simulink model "Lab7_1811"  (R2021b)
settings: Solver=VariableStepAuto  StartTime=0.0  StopTime=10.0  RelTol=1e-3
values from neighbouring files (symbols this model uses):
  a = 1/( 2/norm(r0) - dot(v0,v0)/mu_E )    [Excercise1_2223.m]    (also in Excercise2_2223.m; Lab08_script.m = 42164; Lab7_script.m = 16733.65; Lab7_scriptscalar.m = 16733.65)
  A0 = eye(3)    [Lab08_script.m]    (also in Lab7_script.m; Lab7_scriptscalar.m; Lab_GG.m)
  Area_mb = diag([A1 A2 A3 A4 A5 A6])    [Lab08_script.m]    (also in Lab7_script.m)
  e = horizonsresults(:,2)    [Ex3-5.m]    (also in Excercise1_2223.m = 1/mu_E*cross(v,h)-r./vecnorm(r,2,2); Lab08_script.m = 0; Lab7_script.m = 0.1976; Lab7_scriptscalar.m = 0.1976)
  epsilon = (vecnorm(v,2,2)).^2/2-mu_E./vecnorm(r,2,2)    [Excercise1_2223.m]    (also in Lab08_script.m = deg2rad(23.45); Lab7_script.m = deg2rad(23.45); Lab7_scriptscalar.m = deg2rad(23.45))
  I = [Ix 0 0; 0 Iy 0; 0 0 Iz]    [Lab08_script.m]    (also in Lab7_script.m; Lab7_scriptscalar.m; Lab_GG.m)
  i = horizonsresults(:,3)    [Ex3-5.m]    (also in Lab08_script.m = deg2rad(0); Lab7_script.m = deg2rad(60); Lab7_scriptscalar.m = deg2rad(60); ex3_Lambert.m = kep_arr_M(3))
  I_inv = inv(I)    [Lab08_script.m]    (also in Lab7_script.m; Lab7_scriptscalar.m; Lab_GG.m)
  n = 10    [Chapter3.m]    (also in Lab08_script.m = sqrt(mu_E/(a^3)); Lab7_script.m = sqrt(mu_E/(a^3)); Lab7_scriptscalar.m = sqrt(mu_E/(a^3)); Lab_GG.m = sqrt(mu_E/( R_E+r_orbit)^3))
  N_b_mb = [n1'; n2'; n3'; n4'; n5'; n6']    [Lab08_script.m]    (also in Lab7_script.m)
  n_sun = 2*pi/T_sun    (= 1.99238499086e-07)    [Lab08_script.m]    (also in Lab7_script.m; Lab7_scriptscalar.m)
  r_mb = [base/2 0 0; 0 base/2 0; 0 0 height/2; -base/2 0 0; 0 -base/2 0; 0 0 -height/2]    [Lab08_script.m]
  rho_d_mb = 0.1    [Lab08_script.m]    (also in Lab7_script.m; Lab7_scriptscalar.m)
  rho_s_mb = 0.5    [Lab08_script.m]    (also in Lab7_script.m; Lab7_scriptscalar.m)
  Rs = astroConstants(2)    [Lab08_script.m]    (also in Lab7_script.m; Lab7_scriptscalar.m)
  theta0 = deg2rad(0)    [Lab08_script.m]    (also in Lab7_script.m = deg2rad(230); Lab7_scriptscalar.m = deg2rad(230))
  v1 = [Y1(:,4) Y1(:,5) Y1(:,6)]    [Excercise2_2223.m]    (also in Lab08_script.m = [0 1 -1]'; Lab7_script.m = [0 1 -1]'; Lab7_scriptscalar.m = [0 1 -1]'; Lab_GG.m = [0 1 -1]')
  v2 = [Y2(:,4) Y2(:,5) Y2(:,6)]    [Excercise2_2223.m]    (also in Lab08_script.m = [-1 0 1]'; Lab7_script.m = [-1 0 1]'; Lab7_scriptscalar.m = [-1 0 1]'; Lab_GG.m = [-1 0 1]')
  v3 = [1 -1 0]'    [Lab08_script.m]    (also in Lab7_script.m; Lab7_scriptscalar.m; Lab_GG.m)
libraries: matrix_library x7
settings Model: Creator=sferl  LastModifiedBy=sferl

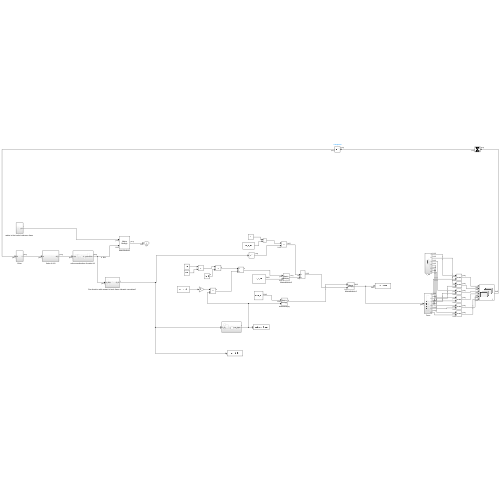
[thumbnail: Simulink's stored preview of the top-level diagram]
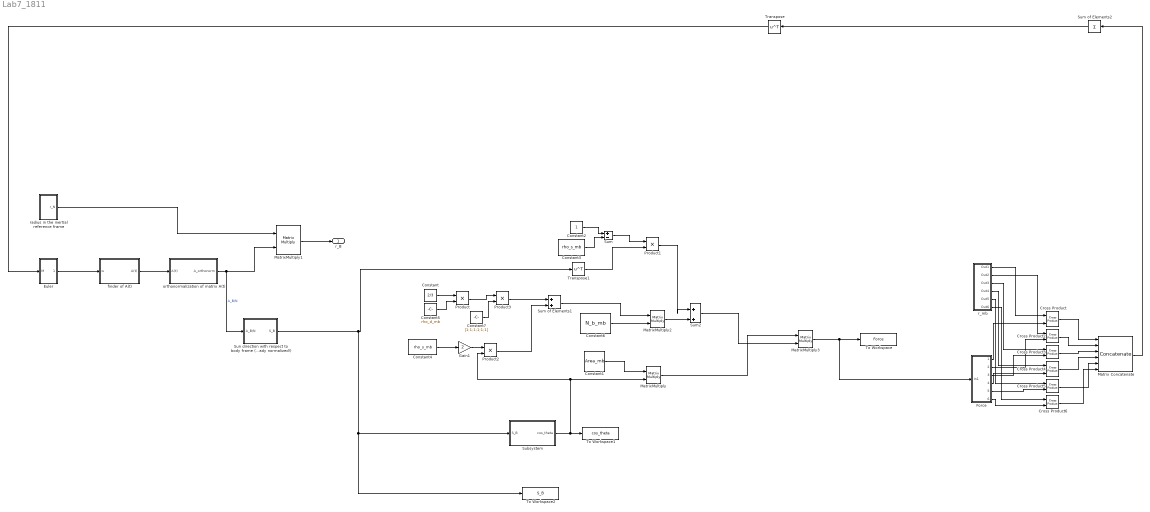
== system Lab7_1811 ==
  Constant : Constant  Value=2/3
  Constant1 : Constant  Value=Area_mb
  Constant2 : Constant
  Constant3 : Constant  Value=rho_s_mb
  Constant4 : Constant  Value=rho_s_mb
  Constant5 : Constant  Value=rho_d_mb
  Constant6 : Constant  Value=N_b_mb
  Constant7 : Constant  Value=[1;1;1;1;1;1]
  Cross Product{,2..6} (6 alike) : matrix_library/Cross Product
      settings: SourceProductBaseCode=SL
  Euler : Subsystem
  Force : Subsystem
  Gain1 : Gain  Gain=2
  Matrix Concatenate : Concatenate  NumInputs=6  Mode=Multidimensional array
  MatrixMultiply{,1..3} (4 alike) : Product  Multiplication=Matrix(*)
  Product{,1..3} (4 alike) : Product
  Subsystem : Subsystem
  Sum : Sum  Inputs=+-
  Sum of Elements1 : Sum
  Sum of Elements2 : Sum  Inputs=+  CollapseMode=Specified dimension
  Sum2 : Sum  Inputs=|++
  Sun direction with respect to body frame (already normalized!) : Subsystem
  To Workspace : ToWorkspace  VariableName=Force  SaveFormat=Timeseries  SampleTime=-1
  To Workspace1 : ToWorkspace  VariableName=cos_theta  SampleTime=-1
  To Workspace2 : ToWorkspace  VariableName=S_B  SampleTime=-1
  Transpose : Math  Operator=transpose  SaturateOnIntegerOverflow=on
  Transpose1 : Math  Operator=transpose  SaturateOnIntegerOverflow=on
  finder of A(t) : Subsystem
  orthonormalization of matrix A(t) : Subsystem
  r_mb : Subsystem
  radius in the inertial reference frame : Subsystem
  r_B : Outport
  wires:
  MatrixMultiply1/1 -> r_B/1
  finder of A(t)/1(A(t)) -> orthonormalization of matrix A(t)/1(A(t))
  orthonormalization of matrix A(t)/1(A_orthonorm) -> Sun direction with respect to body frame (already normalized!)/1(A_B/N), MatrixMultiply1/2  "A_B/N"
  Constant1/1 -> MatrixMultiply/1
  Subsystem/1(cos_theta) -> Product2/2, MatrixMultiply/2, To Workspace1/1
  Constant2/1 -> Sum/1
  Constant3/1 -> Sum/2
  Sum/1 -> Product1/1
  Constant4/1 -> Gain1/1
  Gain1/1 -> Product2/1
  Constant6/1 -> MatrixMultiply2/2
  MatrixMultiply2/1 -> Sum2/2
  Product1/1 -> Sum2/1
  Sum2/1 -> MatrixMultiply3/2
  Transpose1/1 -> Product1/2
  Product/1 -> Product3/1
  Sum of Elements1/1 -> MatrixMultiply2/1
  Constant/1 -> Product/1
  Constant5/1 -> Product/2
  Constant7/1 -> Product3/2
  Product3/1 -> Sum of Elements1/1
  radius in the inertial reference frame/1(r_N) -> MatrixMultiply1/1
  Euler/1(Output1) -> finder of A(t)/1(w)
  Sun direction with respect to body frame (already normalized!)/1(S_B) -> Transpose1/1, Subsystem/1(S_B), To Workspace2/1
  Product2/1 -> Sum of Elements1/2
  MatrixMultiply/1 -> MatrixMultiply3/1
  Cross Product6/1 -> Matrix Concatenate/6
  Cross Product4/1 -> Matrix Concatenate/4
  Cross Product5/1 -> Matrix Concatenate/5
  Cross Product3/1 -> Matrix Concatenate/3
  Matrix Concatenate/1 -> Sum of Elements2/1
  MatrixMultiply3/1 -> Force/1(In1), To Workspace/1
  Cross Product/1 -> Matrix Concatenate/1
  Cross Product2/1 -> Matrix Concatenate/2
  Sum of Elements2/1 -> Transpose/1
  Transpose/1 -> Euler/1(M)
  r_mb/1(Out1) -> Cross Product/1
  r_mb/2(Out2) -> Cross Product2/1
  r_mb/3(Out3) -> Cross Product3/1
  r_mb/4(Out4) -> Cross Product4/1
  r_mb/5(Out5) -> Cross Product5/1
  r_mb/6(Out6) -> Cross Product6/1
  Force/1(Out1) -> Cross Product/2
  Force/2(Out2) -> Cross Product2/2
  Force/3(Out3) -> Cross Product3/2
  Force/4(Out4) -> Cross Product4/2
  Force/5(Out5) -> Cross Product5/2
  Force/6(Out6) -> Cross Product6/2

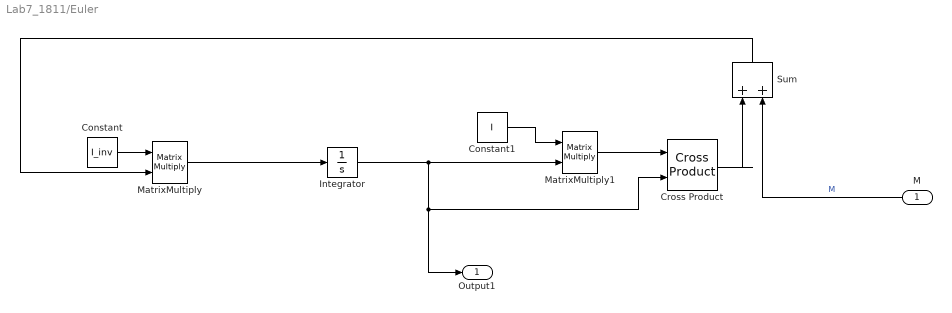
== system Lab7_1811/Euler ==
  M : Inport
  Constant : Constant  Value=I_inv
  Constant1 : Constant  Value=I
  Cross Product : matrix_library/Cross Product
      settings: SourceProductBaseCode=SL
  Integrator : Integrator
  MatrixMultiply : Product  Multiplication=Matrix(*)
  MatrixMultiply1 : Product  Multiplication=Matrix(*)
  Sum : Sum  Inputs=|++
  Output1 : Outport
  wires:
  M/1 -> Sum/2  "M"
  Constant/1 -> MatrixMultiply/1
  MatrixMultiply/1 -> Integrator/1
  Integrator/1 -> Output1/1, Cross Product/2, MatrixMultiply1/2
  Constant1/1 -> MatrixMultiply1/1
  MatrixMultiply1/1 -> Cross Product/1
  Cross Product/1 -> Sum/1
  Sum/1 -> MatrixMultiply/2

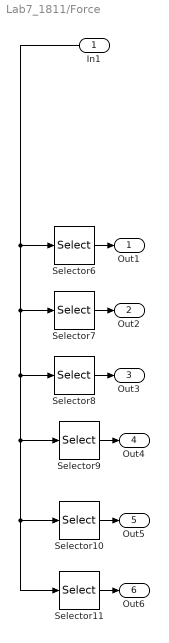
== system Lab7_1811/Force ==
  In1 : Inport
  Selector10 : Selector  NumberOfDimensions=2  InputPortWidth=3  IndexOptions=Starting index (dialog),Starting index (dialog)  Indices=5,1  OutputSizes=1,3
  Selector11 : Selector  NumberOfDimensions=2  InputPortWidth=3  IndexOptions=Starting index (dialog),Starting index (dialog)  Indices=6,1  OutputSizes=1,3
  Selector6 : Selector  NumberOfDimensions=2  InputPortWidth=3  IndexOptions=Starting index (dialog),Starting index (dialog)  Indices=1,1  OutputSizes=1,3
  Selector7 : Selector  NumberOfDimensions=2  InputPortWidth=3  IndexOptions=Starting index (dialog),Starting index (dialog)  Indices=2,1  OutputSizes=1,3
  Selector8 : Selector  NumberOfDimensions=2  InputPortWidth=3  IndexOptions=Starting index (dialog),Starting index (dialog)  Indices=3,1  OutputSizes=1,3
  Selector9 : Selector  NumberOfDimensions=2  InputPortWidth=3  IndexOptions=Starting index (dialog),Starting index (dialog)  Indices=4,1  OutputSizes=1,3
  Out1 : Outport
  Out2 : Outport  Port=2
  Out3 : Outport  Port=3
  Out4 : Outport  Port=4
  Out5 : Outport  Port=5
  Out6 : Outport  Port=6
  wires:
  Selector7/1 -> Out2/1
  Selector6/1 -> Out1/1
  In1/1 -> Selector11/1, Selector10/1, Selector9/1, Selector8/1, Selector7/1, Selector6/1
  Selector9/1 -> Out4/1
  Selector11/1 -> Out6/1
  Selector10/1 -> Out5/1
  Selector8/1 -> Out3/1

== system Lab7_1811/Subsystem ==
  S_B : Inport
  Constant : Constant  Value=N_b_mb
  MatrixMultiply : Product  Multiplication=Matrix(*)
  cos_theta : Outport
  wires:
  Constant/1 -> MatrixMultiply/1
  MatrixMultiply/1 -> cos_theta/1
  S_B/1 -> MatrixMultiply/2

== system Lab7_1811/Sun direction with respect to body frame (already normalized!) ==
  A_B/N : Inport
  Constant7 : Constant  Value=1/Rs
  MatrixMultiply : Product  Multiplication=Matrix(*)
  Product5 : Product
  S_N : Subsystem
  S_B : Outport
  wires:
  S_N/1(Out1) -> MatrixMultiply/2
  A_B/N/1 -> MatrixMultiply/1
  Constant7/1 -> Product5/1
  MatrixMultiply/1 -> Product5/2
  Product5/1 -> S_B/1

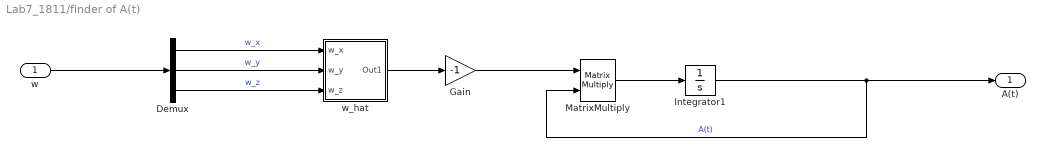
== system Lab7_1811/finder of A(t) ==
  w : Inport
  Demux : Demux  Outputs=3
  Gain : Gain  Gain=-1
  Integrator1 : Integrator  InitialCondition=A0
  MatrixMultiply : Product  Multiplication=Matrix(*)
  w_hat : Subsystem
  A(t) : Outport
  wires:
  w/1 -> Demux/1
  Gain/1 -> MatrixMultiply/1
  Integrator1/1 -> A(t)/1, MatrixMultiply/2  "A(t)"
  w_hat/1(Out1) -> Gain/1
  Demux/3 -> w_hat/3(w_z)  "w_z"
  Demux/2 -> w_hat/2(w_y)  "w_y"
  Demux/1 -> w_hat/1(w_x)  "w_x"
  MatrixMultiply/1 -> Integrator1/1

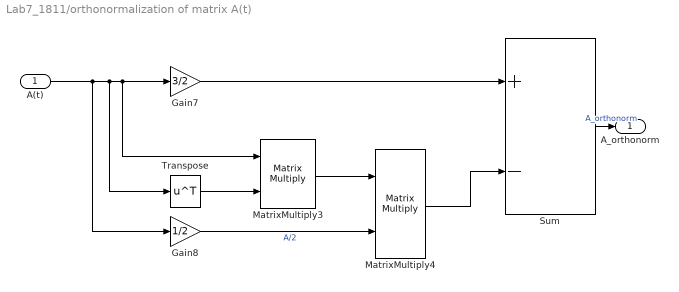
== system Lab7_1811/orthonormalization of matrix A(t) ==
  A(t) : Inport
  Gain7 : Gain  Gain=3/2
  Gain8 : Gain  Gain=1/2
  MatrixMultiply3 : Product  Multiplication=Matrix(*)
  MatrixMultiply4 : Product  Multiplication=Matrix(*)
  Sum : Sum  Inputs=+-
  Transpose : Math  Operator=transpose  SaturateOnIntegerOverflow=on
  A_orthonorm : Outport
  wires:
  Transpose/1 -> MatrixMultiply3/2
  MatrixMultiply4/1 -> Sum/2
  MatrixMultiply3/1 -> MatrixMultiply4/1
  Gain7/1 -> Sum/1
  Gain8/1 -> MatrixMultiply4/2  "A/2"
  A(t)/1 -> Gain8/1, Transpose/1, MatrixMultiply3/1, Gain7/1
  Sum/1 -> A_orthonorm/1  "A_orthonorm"

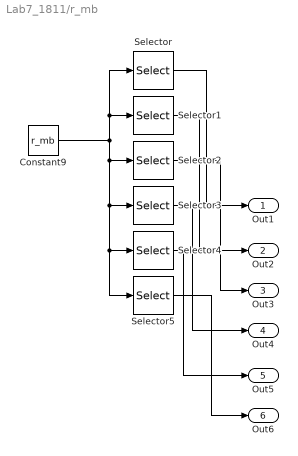
== system Lab7_1811/r_mb ==
  Constant9 : Constant  Value=r_mb
  Selector : Selector  NumberOfDimensions=2  InputPortWidth=3  IndexOptions=Starting index (dialog),Starting index (dialog)  Indices=1,1  OutputSizes=1,3
  Selector1 : Selector  NumberOfDimensions=2  InputPortWidth=3  IndexOptions=Starting index (dialog),Starting index (dialog)  Indices=2,1  OutputSizes=1,3
  Selector2 : Selector  NumberOfDimensions=2  InputPortWidth=3  IndexOptions=Starting index (dialog),Starting index (dialog)  Indices=3,1  OutputSizes=1,3
  Selector3 : Selector  NumberOfDimensions=2  InputPortWidth=3  IndexOptions=Starting index (dialog),Starting index (dialog)  Indices=4,1  OutputSizes=1,3
  Selector4 : Selector  NumberOfDimensions=2  InputPortWidth=3  IndexOptions=Starting index (dialog),Starting index (dialog)  Indices=5,1  OutputSizes=1,3
  Selector5 : Selector  NumberOfDimensions=2  InputPortWidth=3  IndexOptions=Starting index (dialog),Starting index (dialog)  Indices=6,1  OutputSizes=1,3
  Out1 : Outport
  Out2 : Outport  Port=2
  Out3 : Outport  Port=3
  Out4 : Outport  Port=4
  Out5 : Outport  Port=5
  Out6 : Outport  Port=6
  wires:
  Selector4/1 -> Out5/1
  Constant9/1 -> Selector2/1, Selector5/1, Selector4/1, Selector3/1, Selector1/1, Selector/1
  Selector2/1 -> Out3/1
  Selector1/1 -> Out2/1
  Selector/1 -> Out1/1
  Selector3/1 -> Out4/1
  Selector5/1 -> Out6/1

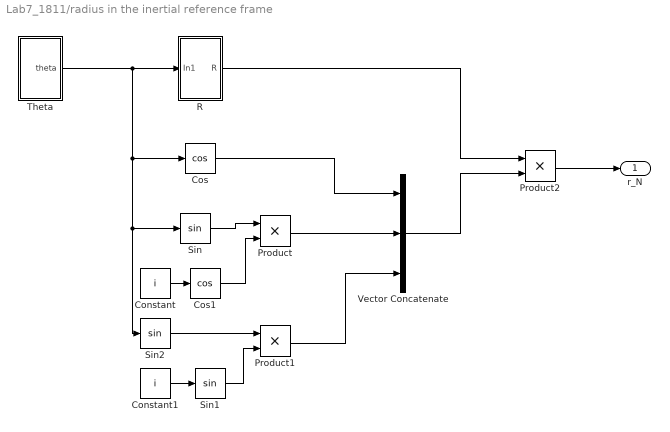
== system Lab7_1811/radius in the inertial reference frame ==
  Constant : Constant  Value=i
  Constant1 : Constant  Value=i
  Cos : Trigonometry  Operator=cos
  Cos1 : Trigonometry  Operator=cos
  Product : Product
  Product1 : Product
  Product2 : Product
  R : Subsystem
  Sin : Trigonometry
  Sin1 : Trigonometry
  Sin2 : Trigonometry
  Theta : Subsystem
  Vector Concatenate : Concatenate  NumInputs=3
  r_N : Outport
  wires:
  Cos/1 -> Vector Concatenate/1
  Theta/1(theta) -> Sin2/1, Sin/1, Cos/1, R/1(In1)
  Constant/1 -> Cos1/1
  Product1/1 -> Vector Concatenate/3
  Sin1/1 -> Product1/2
  Cos1/1 -> Product/2
  R/1(R) -> Product2/1
  Product/1 -> Vector Concatenate/2
  Vector Concatenate/1 -> Product2/2
  Constant1/1 -> Sin1/1
  Sin/1 -> Product/1
  Sin2/1 -> Product1/1
  Product2/1 -> r_N/1

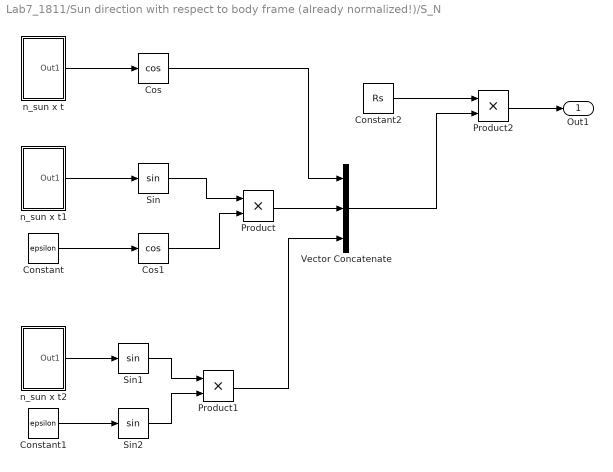
== system Lab7_1811/Sun direction with respect to body frame (already normalized!)/S_N ==
  Constant : Constant  Value=epsilon
  Constant1 : Constant  Value=epsilon
  Constant2 : Constant  Value=Rs
  Cos : Trigonometry  Operator=cos
  Cos1 : Trigonometry  Operator=cos
  Product : Product
  Product1 : Product
  Product2 : Product
  Sin : Trigonometry
  Sin1 : Trigonometry
  Sin2 : Trigonometry
  Vector Concatenate : Concatenate  NumInputs=3
  n_sun x t : Subsystem
  n_sun x t1 : Subsystem
  n_sun x t2 : Subsystem
  Out1 : Outport
  wires:
  n_sun x t2/1(Out1) -> Sin1/1
  Vector Concatenate/1 -> Product2/2
  Sin2/1 -> Product1/2
  Sin/1 -> Product/1
  n_sun x t1/1(Out1) -> Sin/1
  Product1/1 -> Vector Concatenate/3
  Constant2/1 -> Product2/1
  Cos/1 -> Vector Concatenate/1
  Cos1/1 -> Product/2
  Product/1 -> Vector Concatenate/2
  n_sun x t/1(Out1) -> Cos/1
  Constant1/1 -> Sin2/1
  Sin1/1 -> Product1/1
  Constant/1 -> Cos1/1
  Product2/1 -> Out1/1

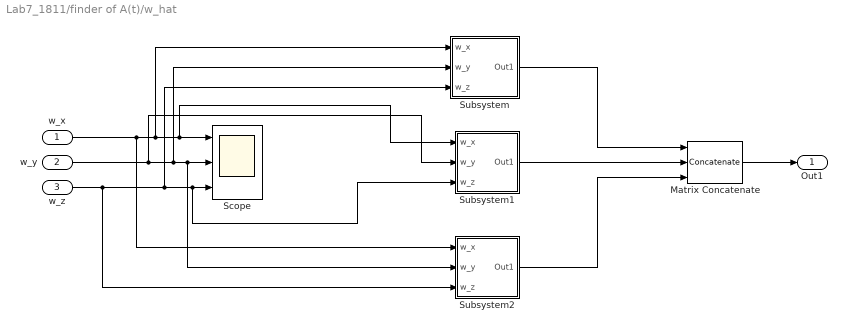
== system Lab7_1811/finder of A(t)/w_hat ==
  w_x : Inport
  w_y : Inport  Port=2
  w_z : Inport  Port=3
  Matrix Concatenate : Concatenate  NumInputs=3  Mode=Multidimensional array  ConcatenateDimension=2
  Scope : Scope  NumInputPorts=3
  Subsystem : Subsystem
  Subsystem1 : Subsystem
  Subsystem2 : Subsystem
  Out1 : Outport
  wires:
  w_y/1 -> Subsystem1/2(w_y), Subsystem/2(w_y), Subsystem2/2(w_y), Scope/2
  w_z/1 -> Subsystem2/3(w_z), Subsystem/3(w_z), Subsystem1/3(w_z), Scope/3
  w_x/1 -> Subsystem2/1(w_x), Subsystem/1(w_x), Subsystem1/1(w_x), Scope/1
  Subsystem2/1(Out1) -> Matrix Concatenate/3
  Subsystem1/1(Out1) -> Matrix Concatenate/2
  Subsystem/1(Out1) -> Matrix Concatenate/1
  Matrix Concatenate/1 -> Out1/1

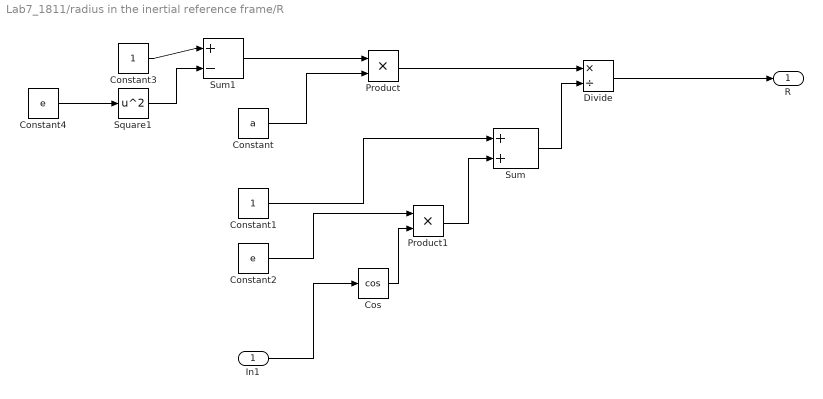
== system Lab7_1811/radius in the inertial reference frame/R ==
  In1 : Inport
  Constant : Constant  Value=a
  Constant1 : Constant
  Constant2 : Constant  Value=e
  Constant3 : Constant
  Constant4 : Constant  Value=e
  Cos : Trigonometry  Operator=cos
  Divide : Product  Inputs=*/
  Product : Product
  Product1 : Product
  Square1 : Math  Operator=square  SaturateOnIntegerOverflow=on
  Sum : Sum  Inputs=|++
  Sum1 : Sum  Inputs=|+-
  R : Outport
  wires:
  Sum/1 -> Divide/2
  Constant1/1 -> Sum/1
  Square1/1 -> Sum1/2
  Product1/1 -> Sum/2
  Constant2/1 -> Product1/1
  Constant/1 -> Product/2
  Divide/1 -> R/1
  Cos/1 -> Product1/2
  Sum1/1 -> Product/1
  In1/1 -> Cos/1
  Constant4/1 -> Square1/1
  Constant3/1 -> Sum1/1
  Product/1 -> Divide/1

== system Lab7_1811/radius in the inertial reference frame/Theta ==
  Denominator : Subsystem
  Divide : Product  Inputs=*/
  Integrator : Integrator  InitialCondition=theta0
  Numerator : Subsystem
  theta : Outport
  wires:
  Numerator/1(Out1) -> Divide/1
  Denominator/1(Output) -> Divide/2
  Integrator/1 -> theta/1, Numerator/1(In1)
  Divide/1 -> Integrator/1

== system Lab7_1811/Sun direction with respect to body frame (already normalized!)/S_N/n_sun x t ==
  Clock : Clock
  Constant : Constant  Value=n_sun
  Product : Product
  Out1 : Outport
  wires:
  Constant/1 -> Product/1
  Clock/1 -> Product/2
  Product/1 -> Out1/1

== system Lab7_1811/Sun direction with respect to body frame (already normalized!)/S_N/n_sun x t1 ==
  Clock : Clock
  Constant : Constant  Value=n_sun
  Product : Product
  Out1 : Outport
  wires:
  Product/1 -> Out1/1
  Clock/1 -> Product/2
  Constant/1 -> Product/1

== system Lab7_1811/Sun direction with respect to body frame (already normalized!)/S_N/n_sun x t2 ==
  Clock : Clock
  Constant : Constant  Value=n_sun
  Product : Product
  Out1 : Outport
  wires:
  Constant/1 -> Product/1
  Clock/1 -> Product/2
  Product/1 -> Out1/1

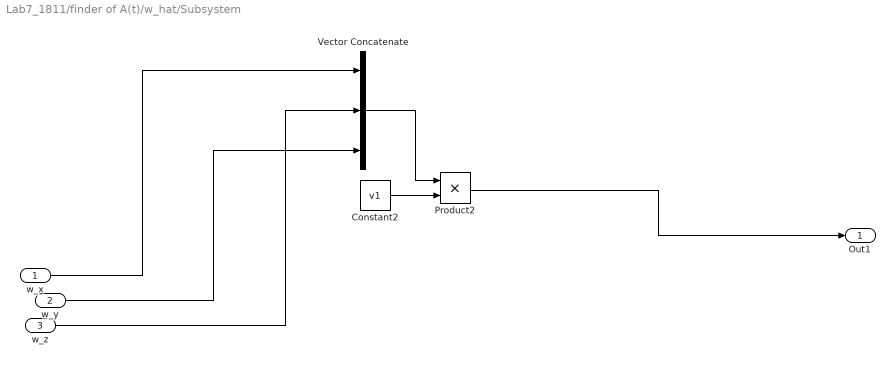
== system Lab7_1811/finder of A(t)/w_hat/Subsystem ==
  w_x : Inport
  w_y : Inport  Port=2
  w_z : Inport  Port=3
  Constant2 : Constant  Value=v1
  Product2 : Product
  Vector Concatenate : Concatenate  NumInputs=3
  Out1 : Outport
  wires:
  Product2/1 -> Out1/1
  Vector Concatenate/1 -> Product2/1
  Constant2/1 -> Product2/2
  w_x/1 -> Vector Concatenate/1
  w_z/1 -> Vector Concatenate/2
  w_y/1 -> Vector Concatenate/3

== system Lab7_1811/finder of A(t)/w_hat/Subsystem1 ==
  w_x : Inport
  w_y : Inport  Port=2
  w_z : Inport  Port=3
  Constant4 : Constant  Value=v2
  Product4 : Product
  Vector Concatenate2 : Concatenate  NumInputs=3
  Out1 : Outport
  wires:
  Constant4/1 -> Product4/2
  Vector Concatenate2/1 -> Product4/1
  Product4/1 -> Out1/1
  w_x/1 -> Vector Concatenate2/3
  w_y/1 -> Vector Concatenate2/2
  w_z/1 -> Vector Concatenate2/1

== system Lab7_1811/finder of A(t)/w_hat/Subsystem2 ==
  w_x : Inport
  w_y : Inport  Port=2
  w_z : Inport  Port=3
  Constant3 : Constant  Value=v3
  Product3 : Product
  Vector Concatenate1 : Concatenate  NumInputs=3
  Out1 : Outport
  wires:
  Product3/1 -> Out1/1
  Constant3/1 -> Product3/2
  w_y/1 -> Vector Concatenate1/1
  Vector Concatenate1/1 -> Product3/1
  w_x/1 -> Vector Concatenate1/2
  w_z/1 -> Vector Concatenate1/3

== system Lab7_1811/radius in the inertial reference frame/Theta/Denominator ==
  Constant3 : Constant
  Constant5 : Constant  Value=3/2
  Power : Math  Operator=pow  SaturateOnIntegerOverflow=on
  Square1 : Math  Operator=square  SaturateOnIntegerOverflow=on
  Sum1 : Sum  Inputs=|+-
  eccentricity : Constant  Value=e
  Output : Outport
  wires:
  Constant3/1 -> Sum1/1
  eccentricity/1 -> Square1/1
  Sum1/1 -> Power/1
  Square1/1 -> Sum1/2
  Constant5/1 -> Power/2
  Power/1 -> Output/1

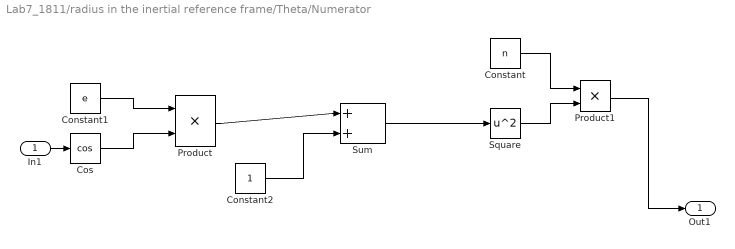
== system Lab7_1811/radius in the inertial reference frame/Theta/Numerator ==
  In1 : Inport
  Constant : Constant  Value=n
  Constant1 : Constant  Value=e
  Constant2 : Constant
  Cos : Trigonometry  Operator=cos
  Product : Product
  Product1 : Product
  Square : Math  Operator=square  SaturateOnIntegerOverflow=on
  Sum : Sum  Inputs=|++
  Out1 : Outport
  wires:
  Constant2/1 -> Sum/2
  Sum/1 -> Square/1
  In1/1 -> Cos/1
  Constant1/1 -> Product/1
  Constant/1 -> Product1/1
  Cos/1 -> Product/2
  Product/1 -> Sum/1
  Square/1 -> Product1/2
  Product1/1 -> Out1/1
